simulink library "Vehicle_Control_Axle2_Battery_Motor2"  (R2026a)
settings: Solver=VariableStepAuto
undefined symbols (not defined in the file): Control
libraries: simulink x4, Damper_Control_Axle2 x2, sl_discontinuities x2, Driveline_Control_Axle2_None x1, Spring_Control_Axle2 x1, Steer_Control_Axle2 x1
Description:
  | Simscape Vehicle Templates Library
  | 
  | Copyright 2018-2026 The MathWorks, Inc.
settings Model: Creator=smiller  LastModifiedBy=smiller

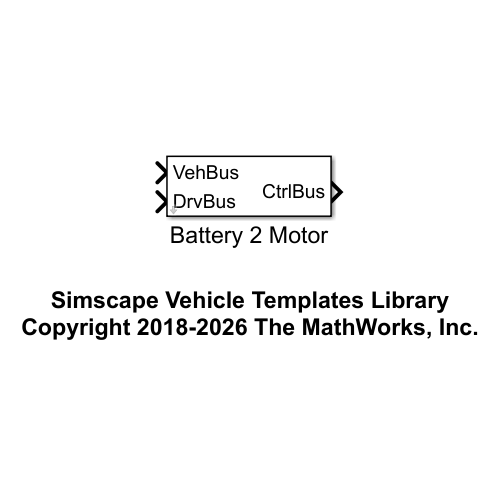
[thumbnail: Simulink's stored preview of the top-level diagram]
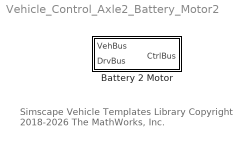
== system Vehicle_Control_Axle2_Battery_Motor2 ==
  note: Simscape Vehicle Templates Library
      | Copyright 2018-2026 The MathWorks, Inc.
  Battery 2 Motor : Subsystem  VariantControl=Battery2Motor  mask(Control of Two Motor Powertrain){ControlElectric=Control.Electric_A1_A2_default, popup_damper_control_A1=None, popup_damper_control_A2=None, popup_spring_control_A1=None, popup_spring_control_A2=None}
      mask prompts: ControlElectric "Control (structure)"; popup_damper_control_A1 "Damper Control Axle 1"; popup_damper_control_A2 "Damper Control Axle 2"; popup_spring_control_A1 "Spring Control Axle 1"; popup_spring_control_A2 "Spring Control Axle 2"
      mask help: Models control algorithm for battery management and regenerative braking of a two motor powertrain.
      mask TypeOptions popup_damper_control_A1: Damper Control/popup_damper_control_A1
      mask TypeOptions popup_damper_control_A2: Damper Control/popup_damper_control_A2
      mask TypeOptions popup_spring_control_A1: Spring Control/popup_spring_control_A1
      mask TypeOptions popup_spring_control_A2: Spring Control/popup_spring_control_A2

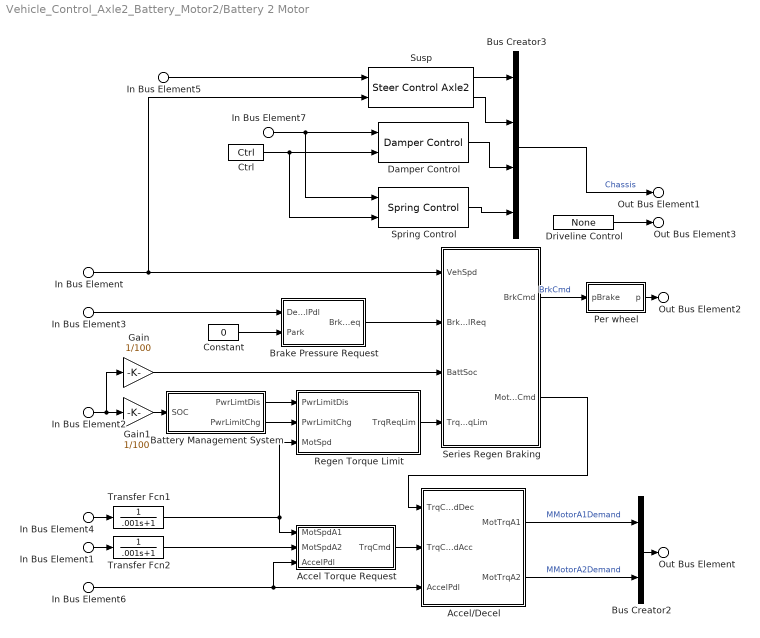
== system Vehicle_Control_Axle2_Battery_Motor2/Battery 2 Motor ==
  In Bus Element7 : Inport  PortName=VehBus
  In Bus Element : Inport  PortName=VehBus  Element=Chassis.Body.CG.vx
  In Bus Element2 : Inport  PortName=VehBus  Element=Power.Battery.SOC
  In Bus Element4 : Inport  PortName=VehBus  Element=Power.MotorA1.w
  In Bus Element1 : Inport  PortName=VehBus  Element=Power.MotorA2.w
  In Bus Element3 : Inport  Port=2  PortName=DrvBus  Element=rBrakePedal
  In Bus Element6 : Inport  Port=2  PortName=DrvBus  Element=rAccelPedal
  In Bus Element5 : Inport  Port=2  PortName=DrvBus  Element=aSteerWheel
  Accel Torque Request : Subsystem
  Accel/Decel : Subsystem
  Battery Management System : Subsystem
  Brake Pressure Request : Subsystem
  Bus Creator2 : BusCreator  Inputs=2
  Bus Creator3 : BusCreator  Inputs=4
  Constant : Constant  Value=0
  Ctrl : Damper_Control_Axle2/Ctrl  SystemSampleTime=-1  VariantActivationTime=update diagram  EmptyChoice=off  PassThrough=off  PassThroughVariantControl=(default)  EmptyChoiceVariantControl=(default)  AllowFlexibleInterface=on  Latency=0  AutoFrameSizeCalculation=off
  Damper Control : Damper_Control_Axle2/Damper Control  VariantControl=Choice  popup_damper_control_A1=None  popup_damper_control_A2=None
  Driveline Control : Driveline_Control_Axle2_None/None  SystemSampleTime=-1  VariantActivationTime=update diagram  EmptyChoice=off  PassThrough=off  PassThroughVariantControl=(default)  EmptyChoiceVariantControl=(default)  AllowFlexibleInterface=on  Latency=0  AutoFrameSizeCalculation=off
  Gain : Gain  Gain=1/100
  Gain1 : Gain  Gain=1/100
  Per wheel : Subsystem
  Regen Torque Limit : Subsystem
  Series Regen Braking : Subsystem  InitFcn=%[~]=autosharedicon('autolibutils',gcb,0);  VariantControl=Variant
  Spring Control : Spring_Control_Axle2/Spring Control  VariantControl=Choice  popup_spring_control_A1=None  popup_gas_spring_A1=Stiff  popup_spring_control_A2=None  popup_gas_spring_A2=Stiff
  Susp : Steer_Control_Axle2/Steer Control Axle2  Steer=ControlElectric.Steer
  Transfer Fcn1 : TransferFcn  Denominator=[.001 1]
  Transfer Fcn2 : TransferFcn  Denominator=[.001 1]
  Out Bus Element : Outport  PortName=CtrlBus  Element=Power
  Out Bus Element2 : Outport  PortName=CtrlBus  Element=Brakes
  Out Bus Element1 : Outport  PortName=CtrlBus  Element=Chassis
  Out Bus Element3 : Outport  PortName=CtrlBus  Element=Driveline
  wires:
  In Bus Element/1 -> Series Regen Braking/1(VehSpd), Susp/2
  In Bus Element5/1 -> Susp/1
  Transfer Fcn2/1 -> Accel Torque Request/2(MotSpdA2)
  In Bus Element1/1 -> Transfer Fcn2/1
  Battery Management System/1(PwrLimtDis) -> Regen Torque Limit/1(PwrLimitDis)
  Battery Management System/2(PwrLimitChg) -> Regen Torque Limit/2("PwrLimitChg ")
  Transfer Fcn1/1 -> Accel Torque Request/1(MotSpdA1), Regen Torque Limit/3(MotSpd)
  In Bus Element6/1 -> Accel Torque Request/3(AccelPdl), Accel/Decel/3(AccelPdl)
  Accel Torque Request/1(TrqCmd) -> Accel/Decel/2(TrqCmdAcc)
  Series Regen Braking/2(" MotTrqCmd") -> Accel/Decel/1(TrqCmdDec)
  Regen Torque Limit/1("TrqReqLim ") -> Series Regen Braking/4(TrqReqLim)
  Accel/Decel/2(MotTrqA2) -> Bus Creator2/2  "MMotorA2Demand"
  Accel/Decel/1(MotTrqA1) -> Bus Creator2/1  "MMotorA1Demand"
  Constant/1 -> Brake Pressure Request/2(Park)
  Gain1/1 -> Battery Management System/1(SOC)
  In Bus Element4/1 -> Transfer Fcn1/1
  Brake Pressure Request/1(BrkDecelReq) -> Series Regen Braking/2(BrkDecelReq)
  Gain/1 -> Series Regen Braking/3(BattSoc)
  In Bus Element3/1 -> Brake Pressure Request/1(DecelPdl)
  In Bus Element2/1 -> Gain/1, Gain1/1
  Series Regen Braking/1(" BrkCmd") -> Per wheel/1(pBrake)  "BrkCmd"
  Bus Creator2/1 -> Out Bus Element/1
  Damper Control/1 -> Bus Creator3/3
  Susp/1 -> Bus Creator3/1
  Bus Creator3/1 -> Out Bus Element1/1  "Chassis"
  Spring Control/1 -> Bus Creator3/4
  Susp/2 -> Bus Creator3/2
  Driveline Control/1 -> Out Bus Element3/1
  Per wheel/1(p) -> Out Bus Element2/1
  In Bus Element7/1 -> Spring Control/1, Damper Control/1
  Ctrl/1 -> Spring Control/2, Damper Control/2

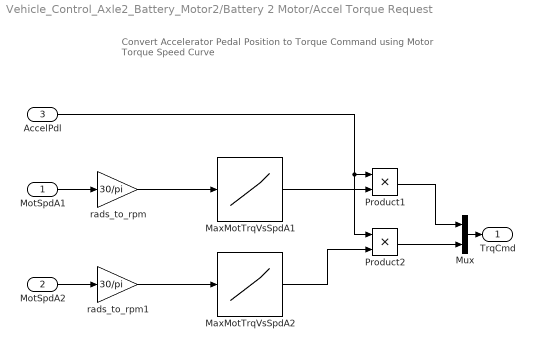
== system Vehicle_Control_Axle2_Battery_Motor2/Battery 2 Motor/Accel Torque Request ==
  note: Convert Accelerator Pedal Position to Torque Command
      | using Motor Torque Speed Curve
  MotSpdA1 : Inport
  MotSpdA2 : Inport  Port=2
  AccelPdl : Inport  Port=3
  MaxMotTrqVsSpdA1 : Lookup_n-D  NumberOfTableDimensions=1  BreakpointsForDimension1=ControlElectric.MotorA1.TorqueSpd.w.Value %Mot.w_eff_bp_EV_rear  Table=ControlElectric.MotorA1.TorqueSpd.trq.Value % Mot.T_t_EV_rear  ExtrapMethod=Clip  UseLastTableValue=on  InternalRulePriority=Speed  OutDataTypeStr=Inherit: Inherit from 'Table data'  RndMeth=Simplest
  MaxMotTrqVsSpdA2 : Lookup_n-D  NumberOfTableDimensions=1  BreakpointsForDimension1=ControlElectric.MotorA2.TorqueSpd.w.Value  Table=ControlElectric.MotorA2.TorqueSpd.trq.Value  ExtrapMethod=Clip  UseLastTableValue=on  InternalRulePriority=Speed  OutDataTypeStr=Inherit: Inherit from 'Table data'  RndMeth=Simplest
  Mux : Mux  Inputs=2
  Product1 : Product
  Product2 : Product
  rads_to_rpm : Gain  Gain=30/pi
  rads_to_rpm1 : Gain  Gain=30/pi
  TrqCmd : Outport  VectorParamsAs1DForOutWhenUnconnected=off
  wires:
  Mux/1 -> TrqCmd/1
  Product2/1 -> Mux/2
  MaxMotTrqVsSpdA2/1 -> Product2/2
  rads_to_rpm1/1 -> MaxMotTrqVsSpdA2/1
  MotSpdA2/1 -> rads_to_rpm1/1
  Product1/1 -> Mux/1
  MaxMotTrqVsSpdA1/1 -> Product1/2
  AccelPdl/1 -> Product2/1, Product1/1
  MotSpdA1/1 -> rads_to_rpm/1
  rads_to_rpm/1 -> MaxMotTrqVsSpdA1/1

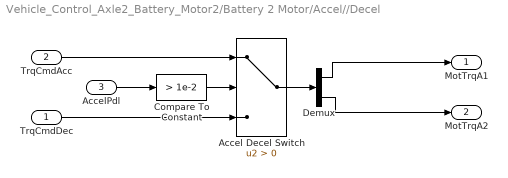
== system Vehicle_Control_Axle2_Battery_Motor2/Battery 2 Motor/Accel//Decel ==
  TrqCmdDec : Inport
  TrqCmdAcc : Inport  Port=2
  AccelPdl : Inport  Port=3
  Accel Decel Switch : Switch  Criteria=u2 > Threshold  SaturateOnIntegerOverflow=off  InputSameDT=off
  Compare To Constant : simulink/Logic and Bit Operations/Compare To Constant  relop=>  const=1e-2  OutDataTypeStr=boolean  ZeroCross=off
  Demux : Demux  Outputs=2
  MotTrqA1 : Outport  VectorParamsAs1DForOutWhenUnconnected=off
  MotTrqA2 : Outport  Port=2  VectorParamsAs1DForOutWhenUnconnected=off
  wires:
  Demux/2 -> MotTrqA2/1
  Demux/1 -> MotTrqA1/1
  Compare To Constant/1 -> Accel Decel Switch/2
  AccelPdl/1 -> Compare To Constant/1
  TrqCmdAcc/1 -> Accel Decel Switch/1
  Accel Decel Switch/1 -> Demux/1
  TrqCmdDec/1 -> Accel Decel Switch/3

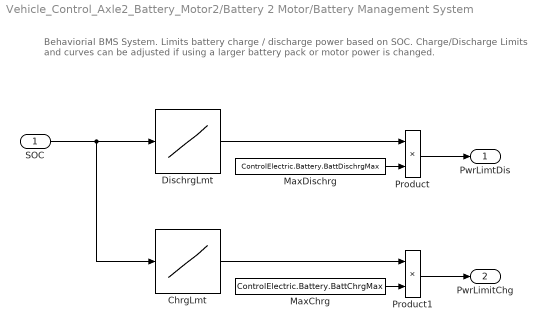
== system Vehicle_Control_Axle2_Battery_Motor2/Battery 2 Motor/Battery Management System ==
  note: Behaviorial BMS System. Limits battery charge / discharge power based on SOC.
      |
      | Charge/Discharge Limits and curves can be adjusted if using a larger battery pack
      | or motor power is changed.
  SOC : Inport
  ChrgLmt : Lookup_n-D  NumberOfTableDimensions=1  BreakpointsForDimension1=ControlElectric.Battery.SOC_bpt  Table=ControlElectric.Battery.ChrgLmt_bpt  ExtrapMethod=Clip  UseLastTableValue=on  InternalRulePriority=Speed  RndMeth=Simplest
  DischrgLmt : Lookup_n-D  NumberOfTableDimensions=1  BreakpointsForDimension1=ControlElectric.Battery.SOC_bpt  Table=ControlElectric.Battery.DischrgLmt_bpt  ExtrapMethod=Clip  UseLastTableValue=on  InternalRulePriority=Speed  RndMeth=Simplest
  MaxChrg : Constant  Value=ControlElectric.Battery.BattChrgMax
  MaxDischrg : Constant  Value=ControlElectric.Battery.BattDischrgMax
  Product : Product
  Product1 : Product
  PwrLimtDis : Outport  VectorParamsAs1DForOutWhenUnconnected=off
  PwrLimitChg : Outport  Port=2  VectorParamsAs1DForOutWhenUnconnected=off
  wires:
  SOC/1 -> DischrgLmt/1, ChrgLmt/1
  MaxChrg/1 -> Product1/2
  MaxDischrg/1 -> Product/2
  Product/1 -> PwrLimtDis/1
  Product1/1 -> PwrLimitChg/1
  ChrgLmt/1 -> Product1/1
  DischrgLmt/1 -> Product/1

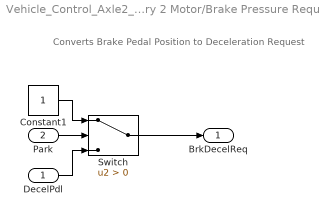
== system Vehicle_Control_Axle2_Battery_Motor2/Battery 2 Motor/Brake Pressure Request ==
  note: Converts Brake Pedal Position to Deceleration Request
  DecelPdl : Inport
  Park : Inport  Port=2
  Constant1 : Constant
  Switch : Switch  Criteria=u2 > Threshold  ZeroCross=off  SaturateOnIntegerOverflow=off  InputSameDT=off
  BrkDecelReq : Outport  VectorParamsAs1DForOutWhenUnconnected=off
  wires:
  DecelPdl/1 -> Switch/3
  Constant1/1 -> Switch/1
  Switch/1 -> BrkDecelReq/1
  Park/1 -> Switch/2

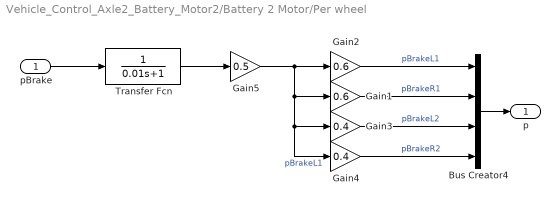
== system Vehicle_Control_Axle2_Battery_Motor2/Battery 2 Motor/Per wheel ==
  pBrake : Inport
  Bus Creator4 : BusCreator  Inputs=4
  Gain1 : Gain  Gain=0.6
  Gain2 : Gain  Gain=0.6
  Gain3 : Gain  Gain=0.4
  Gain4 : Gain  Gain=0.4
  Gain5 : Gain  Gain=0.5
  Transfer Fcn : TransferFcn  Denominator=[0.01 1]
  p : Outport  VectorParamsAs1DForOutWhenUnconnected=off
  wires:
  Transfer Fcn/1 -> Gain5/1
  Gain5/1 -> Gain4/1, Gain3/1, Gain1/1, Gain2/1  "pBrakeL1"
  Gain2/1 -> Bus Creator4/1  "pBrakeL1"
  pBrake/1 -> Transfer Fcn/1
  Bus Creator4/1 -> p/1
  Gain1/1 -> Bus Creator4/2  "pBrakeR1"
  Gain3/1 -> Bus Creator4/3  "pBrakeL2"
  Gain4/1 -> Bus Creator4/4  "pBrakeR2"

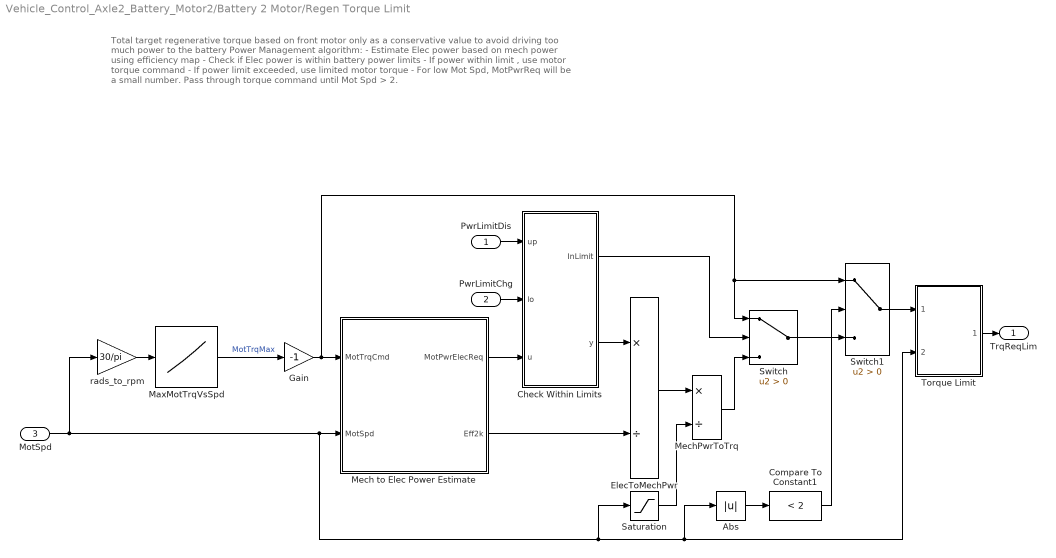
== system Vehicle_Control_Axle2_Battery_Motor2/Battery 2 Motor/Regen Torque Limit ==
  note: Total target regenerative torque based on front motor only as a conservative value to avoid driving too much power to the battery
      |
      | Power Management algorithm:
      | - Estimate Elec power based on mech power using efficiency map
      | - Check if Elec power is within battery power limits
      | - If power within limit , use motor torque command
      | - If power limit exceeded, use limited motor torque
      | - For low Mot Spd, MotPwrReq will be a small number.  Pass through torque command until Mot Spd > 2.
  PwrLimitDis : Inport
  "PwrLimitChg " : Inport  Port=2
  MotSpd : Inport  Port=3
  Abs : Abs  ZeroCross=off  SaturateOnIntegerOverflow=off
  Check Within Limits : Subsystem
  Compare To Constant1 : simulink/Logic and Bit Operations/Compare To Constant  relop=<  const=2  OutDataTypeStr=boolean  ZeroCross=off
  ElecToMechPwr : Product  Inputs=*/
  Gain : Gain  Gain=-1
  MaxMotTrqVsSpd : Lookup_n-D  NumberOfTableDimensions=1  BreakpointsForDimension1=ControlElectric.MotorA1.TorqueSpd.w.Value  Table=ControlElectric.MotorA1.TorqueSpd.trq.Value  ExtrapMethod=Clip  UseLastTableValue=on  InternalRulePriority=Speed  OutDataTypeStr=Inherit: Inherit from 'Table data'  RndMeth=Simplest
  Mech to Elec Power Estimate : Subsystem
  MechPwrToTrq : Product  Inputs=*/
  Saturation : Saturate  UpperLimit=inf  LowerLimit=2
  Switch : Switch  Criteria=u2 > Threshold  ZeroCross=off  SaturateOnIntegerOverflow=off  InputSameDT=off
  Switch1 : Switch  Criteria=u2 > Threshold  ZeroCross=off  SaturateOnIntegerOverflow=off  InputSameDT=off
  Torque Limit : Subsystem
  rads_to_rpm : Gain  Gain=30/pi
  "TrqReqLim " : Outport  VectorParamsAs1DForOutWhenUnconnected=off
  wires:
  MotSpd/1 -> rads_to_rpm/1, Mech to Elec Power Estimate/2(MotSpd), Saturation/1, Abs/1, Torque Limit/2(MotSpd)
  MaxMotTrqVsSpd/1 -> Gain/1  "MotTrqMax"
  rads_to_rpm/1 -> MaxMotTrqVsSpd/1
  ElecToMechPwr/1 -> MechPwrToTrq/1
  MechPwrToTrq/1 -> Switch/3
  Saturation/1 -> MechPwrToTrq/2
  Compare To Constant1/1 -> Switch1/2
  Abs/1 -> Compare To Constant1/1
  Switch/1 -> Switch1/3
  Mech to Elec Power Estimate/1(MotPwrElecReq) -> Check Within Limits/3(u)
  Check Within Limits/2(y) -> ElecToMechPwr/1
  Check Within Limits/1(InLimit) -> Switch/2
  Gain/1 -> Switch1/1, Switch/1, Mech to Elec Power Estimate/1(MotTrqCmd)
  "PwrLimitChg "/1 -> Check Within Limits/2(lo)
  PwrLimitDis/1 -> Check Within Limits/1(up)
  Mech to Elec Power Estimate/2(Eff2k) -> ElecToMechPwr/2
  Torque Limit/1(MotReqCmd) -> "TrqReqLim "/1
  Switch1/1 -> Torque Limit/1(MotTrq)

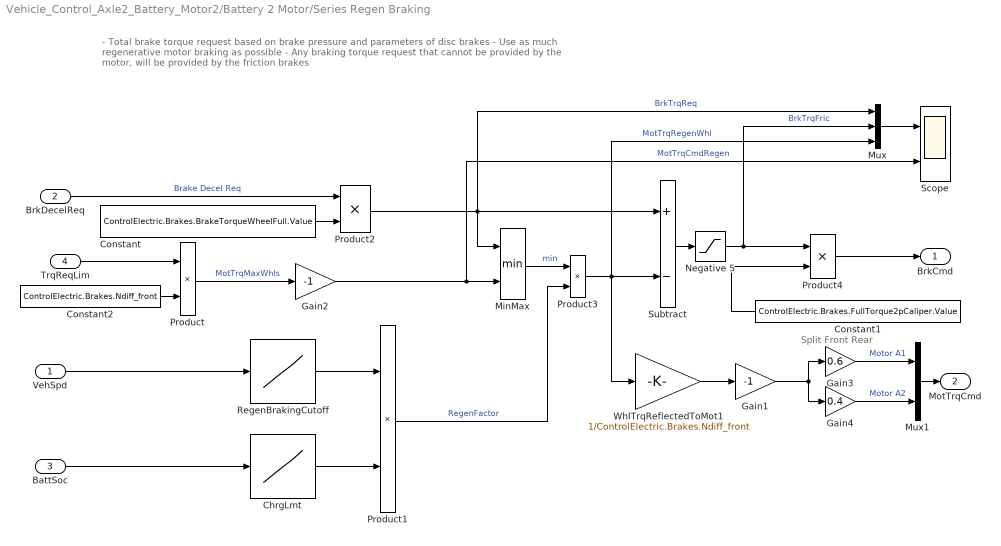
== system Vehicle_Control_Axle2_Battery_Motor2/Battery 2 Motor/Series Regen Braking ==
  note: - Total brake torque request based on brake pressure and parameters of disc brakes
      | - Use as much regenerative motor braking as possible
      | - Any braking torque request that cannot be provided by the motor, will be provided by the friction brakes
  note: Split Front Rear
  VehSpd : Inport
  BrkDecelReq : Inport  Port=2
  BattSoc : Inport  Port=3
  TrqReqLim : Inport  Port=4
  ChrgLmt : Lookup_n-D  NumberOfTableDimensions=1  BreakpointsForDimension1=ControlElectric.Battery.SOC_bpt  Table=ControlElectric.Battery.ChrgLmt_bpt  ExtrapMethod=Clip  UseLastTableValue=on  InternalRulePriority=Speed  RndMeth=Simplest
  Constant : Constant  Value=ControlElectric.Brakes.BrakeTorqueWheelFull.Value
  Constant1 : Constant  Value=ControlElectric.Brakes.FullTorque2pCaliper.Value
  Constant2 : Constant  Value=ControlElectric.Brakes.Ndiff_front
  Gain1 : Gain  Gain=-1
  Gain2 : Gain  Gain=-1
  Gain3 : Gain  Gain=0.6
  Gain4 : Gain  Gain=0.4
  MinMax : MinMax  Inputs=2
  Mux : Mux  Inputs=3
  Mux1 : Mux  Inputs=2
  Negative 5 : Saturate  UpperLimit=inf  LowerLimit=0  ZeroCross=off
  Product{,1..3} (4 alike) : Product
  Product4 : Product  Inputs=**
  RegenBrakingCutoff : Lookup_n-D  NumberOfTableDimensions=1  BreakpointsForDimension1=ControlElectric.Power.RegenBrkSpd_bpt  Table=ControlElectric.Power.RegenBrkCutOff  ExtrapMethod=Clip  UseLastTableValue=on  InternalRulePriority=Speed  RndMeth=Simplest
  Scope : Scope  NumInputPorts=2
      settings: ActiveDisplayYMinimum=-294.72625  ActiveDisplayYMaximum=2652.53625
  Subtract : Sum  Inputs=+-
  WhlTrqReflectedToMot1 : Gain  Gain=1/ControlElectric.Brakes.Ndiff_front
  " BrkCmd" : Outport  VectorParamsAs1DForOutWhenUnconnected=off
  " MotTrqCmd" : Outport  Port=2  VectorParamsAs1DForOutWhenUnconnected=off
  wires:
  Constant2/1 -> Product/2
  Mux1/1 -> " MotTrqCmd"/1
  Gain4/1 -> Mux1/2  "Motor A2"
  Gain3/1 -> Mux1/1  "Motor A1"
  Product/1 -> Gain2/1  "MotTrqMaxWhls"
  Gain2/1 -> Scope/2, MinMax/2  "MotTrqCmdRegen"
  Gain1/1 -> Gain4/1, Gain3/1
  WhlTrqReflectedToMot1/1 -> Gain1/1
  TrqReqLim/1 -> Product/1
  Mux/1 -> Scope/1
  Product3/1 -> Mux/3, Subtract/2, WhlTrqReflectedToMot1/1  "MotTrqRegenWhl"
  Constant1/1 -> Product4/2
  Constant/1 -> Product2/2
  BrkDecelReq/1 -> Product2/1  "Brake Decel Req"
  Product2/1 -> Mux/1, Subtract/1, MinMax/1  "BrkTrqReq"
  MinMax/1 -> Product3/1  "min"
  ChrgLmt/1 -> Product1/2
  VehSpd/1 -> RegenBrakingCutoff/1
  RegenBrakingCutoff/1 -> Product1/1
  Product1/1 -> Product3/2  "RegenFactor"
  Subtract/1 -> Negative 5/1
  BattSoc/1 -> ChrgLmt/1
  Negative 5/1 -> Mux/2, Product4/1  "BrkTrqFric"
  Product4/1 -> " BrkCmd"/1

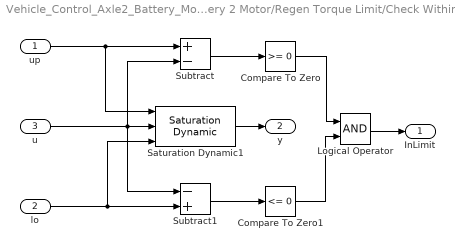
== system Vehicle_Control_Axle2_Battery_Motor2/Battery 2 Motor/Regen Torque Limit/Check Within Limits ==
  up : Inport
  lo : Inport  Port=2
  u : Inport  Port=3
  Compare To Zero : simulink/Logic and Bit Operations/Compare To Zero  relop=>=  OutDataTypeStr=boolean
  Compare To Zero1 : simulink/Logic and Bit Operations/Compare To Zero  relop=<=  OutDataTypeStr=boolean
  Logical Operator : Logic  AllPortsSameDT=off  OutDataTypeStr=boolean
  Saturation Dynamic1 : sl_discontinuities/Saturation Dynamic  OutMin=[]  OutMax=[]  OutDataTypeStr=Inherit: Same as second input  OutDataType=fixdt(1, 16)  OutScaling=2^-10  DoSatur=off
  Subtract : Sum  Inputs=+-
  Subtract1 : Sum  Inputs=-+
  InLimit : Outport  SampleTime=0  VectorParamsAs1DForOutWhenUnconnected=off
  y : Outport  Port=2  VectorParamsAs1DForOutWhenUnconnected=off
  wires:
  Saturation Dynamic1/1 -> y/1
  lo/1 -> Subtract1/2, Saturation Dynamic1/3
  up/1 -> Subtract/1, Saturation Dynamic1/1
  u/1 -> Subtract1/1, Subtract/2, Saturation Dynamic1/2
  Subtract/1 -> Compare To Zero/1
  Subtract1/1 -> Compare To Zero1/1
  Compare To Zero/1 -> Logical Operator/1
  Compare To Zero1/1 -> Logical Operator/2
  Logical Operator/1 -> InLimit/1

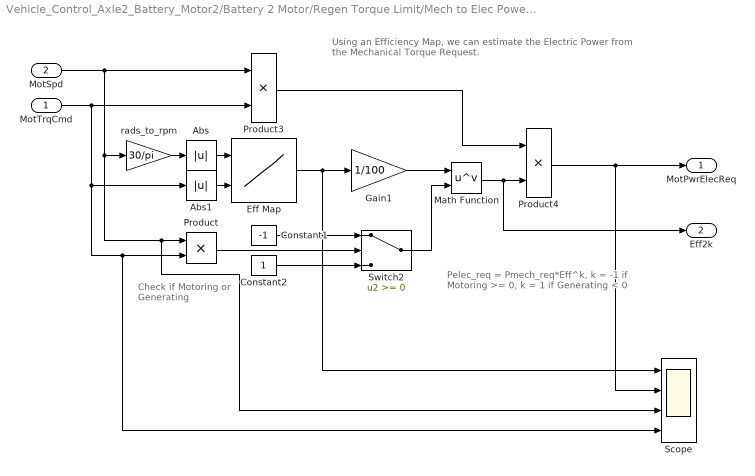
== system Vehicle_Control_Axle2_Battery_Motor2/Battery 2 Motor/Regen Torque Limit/Mech to Elec Power Estimate ==
  note: Check if Motoring
      | or Generating
  note: Using an Efficiency Map, we can estimate the
      | Electric Power from the Mechanical  Torque Request.
  note: Pelec_req = Pmech_req*Eff^k,
      | k = -1 if Motoring >= 0,
      | k = 1 if Generating < 0
  MotTrqCmd : Inport
  MotSpd : Inport  Port=2
  Abs : Abs  ZeroCross=off  SaturateOnIntegerOverflow=off
  Abs1 : Abs  ZeroCross=off  SaturateOnIntegerOverflow=off
  Constant1 : Constant  Value=-1  SampleTime=0
  Constant2 : Constant  SampleTime=0
  Eff Map : Lookup_n-D  BreakpointsForDimension1=ControlElectric.MotorA1.LossTable.w.Value  BreakpointsForDimension2=ControlElectric.MotorA1.LossTable.trq.Value  Table=ControlElectric.MotorA1.LossTable.efficiency.Value  ExtrapMethod=Clip  UseLastTableValue=on  InternalRulePriority=Speed  OutDataTypeStr=Inherit: Inherit from 'Table data'  RndMeth=Simplest
      settings: InputPortMap=u0,u1
  Gain1 : Gain  Gain=1/100
  Math Function : Math  Operator=pow  SignedPower=on  OutputSignalType=real
  Product : Product
  Product3 : Product
  Product4 : Product
  Scope : Scope  NumInputPorts=4
      settings: ActiveDisplayYMinimum=84.125  ActiveDisplayYMaximum=92.875  DataLoggingVariableName=ScopeData2
  Switch2 : Switch  ZeroCross=off  SaturateOnIntegerOverflow=off  InputSameDT=off
  rads_to_rpm : Gain  Gain=30/pi
  MotPwrElecReq : Outport  VectorParamsAs1DForOutWhenUnconnected=off
  Eff2k : Outport  Port=2  VectorParamsAs1DForOutWhenUnconnected=off
  wires:
  Product3/1 -> Product4/1
  Switch2/1 -> Math Function/2
  Constant1/1 -> Switch2/1
  Constant2/1 -> Switch2/3
  Eff Map/1 -> Gain1/1, Scope/1
  Abs/1 -> Eff Map/1
  Gain1/1 -> Math Function/1
  Math Function/1 -> Eff2k/1, Product4/2
  Product4/1 -> MotPwrElecReq/1, Scope/2
  Abs1/1 -> Eff Map/2
  rads_to_rpm/1 -> Abs/1
  Product/1 -> Switch2/2
  MotSpd/1 -> Product3/1, Product/1, Scope/3, rads_to_rpm/1
  MotTrqCmd/1 -> Product3/2, Scope/4, Product/2, Abs1/1

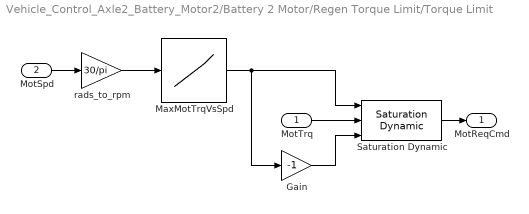
== system Vehicle_Control_Axle2_Battery_Motor2/Battery 2 Motor/Regen Torque Limit/Torque Limit ==
  MotTrq : Inport
  MotSpd : Inport  Port=2
  Gain : Gain  Gain=-1
  MaxMotTrqVsSpd : Lookup_n-D  NumberOfTableDimensions=1  BreakpointsForDimension1=ControlElectric.MotorA1.TorqueSpd.w.Value  Table=ControlElectric.MotorA1.TorqueSpd.trq.Value  ExtrapMethod=Clip  UseLastTableValue=on  InternalRulePriority=Speed  OutDataTypeStr=Inherit: Inherit from 'Table data'  RndMeth=Simplest
  Saturation Dynamic : sl_discontinuities/Saturation Dynamic  OutMin=[]  OutMax=[]  OutDataTypeStr=Inherit: Same as second input  OutDataType=fixdt(1, 16)  OutScaling=2^-10  DoSatur=off
  rads_to_rpm : Gain  Gain=30/pi
  MotReqCmd : Outport  VectorParamsAs1DForOutWhenUnconnected=off
  wires:
  MotTrq/1 -> Saturation Dynamic/2
  MotSpd/1 -> rads_to_rpm/1
  MaxMotTrqVsSpd/1 -> Gain/1, Saturation Dynamic/1
  rads_to_rpm/1 -> MaxMotTrqVsSpd/1
  Gain/1 -> Saturation Dynamic/3
  Saturation Dynamic/1 -> MotReqCmd/1
